simulink library "VoidTrackerDerivates"  (R2021a)
settings: Solver=VariableStepAuto  StartTime=0.0  StopTime=10.0  RelTol=1e-3
settings Model: Creator=z_zha  LastModifiedBy=z_zha

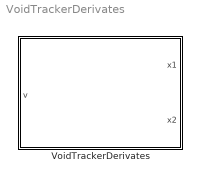
== system VoidTrackerDerivates ==
  VoidTrackerDerivates : Subsystem  mask{R=300, a1=1, b1=1, a2=1, b2=1}
      mask prompts: R "Velocity coffeicient 'R'"; a1 "Err-function parameter 'a'(Named 'a1')"; b1 "Err-function parameter 'b'(Named 'b1')"; a2 "DTrack-function parameter 'a'(Named 'a2')"; b2 "DTrack-function parameter 'b'(Named 'b2')"

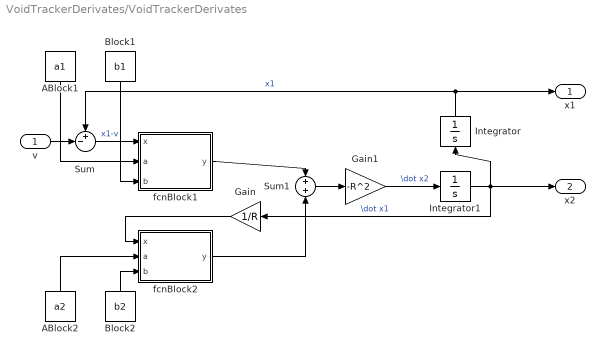
== system VoidTrackerDerivates/VoidTrackerDerivates ==
  v : Inport
  ABlock1 : Constant  Value=a1
  ABlock2 : Constant  Value=a2
  Block1 : Constant  Value=b1
  Block2 : Constant  Value=b2
  Gain : Gain  Gain=1/R
  Gain1 : Gain  Gain=-R^2
  Integrator : Integrator
  Integrator1 : Integrator
  Sum : Sum  Inputs=+-|
  Sum1 : Sum  Inputs=+|+
  fcnBlock1 : MATLAB Function  TreatAsAtomicUnit=on
  fcnBlock2 : MATLAB Function  TreatAsAtomicUnit=on
  x1 : Outport  VectorParamsAs1DForOutWhenUnconnected=off
  x2 : Outport  Port=2  VectorParamsAs1DForOutWhenUnconnected=off
  wires:
  v/1 -> Sum/2
  Integrator/1 -> Sum/1, x1/1  "x1"
  ABlock2/1 -> fcnBlock2/2(a)
  Block1/1 -> fcnBlock1/3(b)
  Sum1/1 -> Gain1/1
  Block2/1 -> fcnBlock2/3(b)
  Sum/1 -> fcnBlock1/1(x)  "x1-v"
  Integrator1/1 -> Gain/1, Integrator/1, x2/1  "\\dot x1"
  ABlock1/1 -> fcnBlock1/2(a)
  Gain1/1 -> Integrator1/1  "\\dot x2"
  fcnBlock1/1(y) -> Sum1/1
  fcnBlock2/1(y) -> Sum1/2
  Gain/1 -> fcnBlock2/1(x)

== matlab function VoidTrackerDerivates/fcnBlock2 ==
  data: x input; y output; a input; b input
function y = fcn(x, a, b)
y=1;

== matlab function VoidTrackerDerivates/fcnBlock1 ==
  data: x input; y output; a input; b input
function y = fcn(x, a, b) 
y = 1;
